simulink subsystem "motores"  (R2023b)
settings: Solver=VariableStepAuto  StartTime=0.0  StopTime=10.0  RelTol=1e-3
libraries: arduinolib x6, simulink x2
settings Model: Creator=Usuario_UMA  LastModifiedBy=Manuel

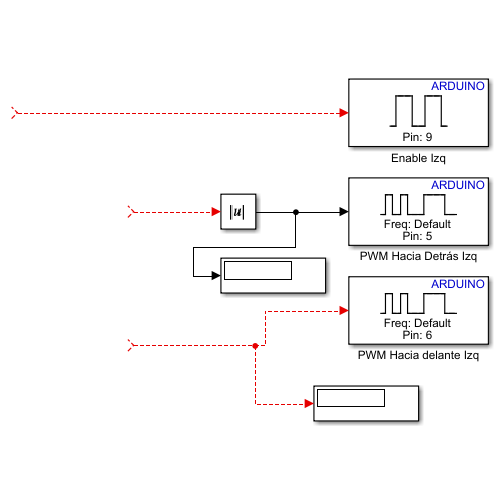
[thumbnail: Simulink's stored preview of the top-level diagram]
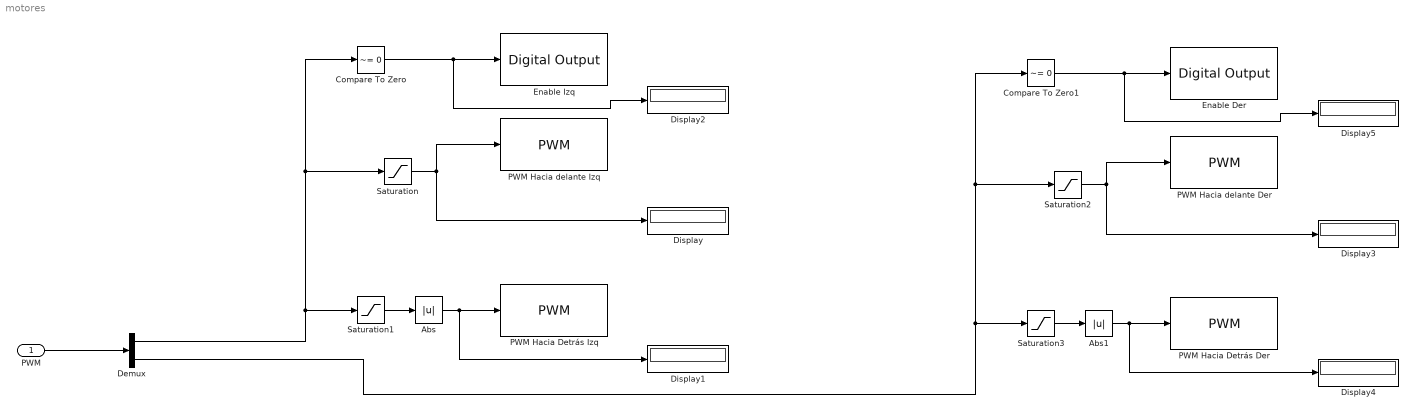
== system motores ==
  PWM : Inport
  Abs : Abs  SaturateOnIntegerOverflow=off
  Abs1 : Abs  SaturateOnIntegerOverflow=off
  Compare To Zero : simulink/Logic and Bit Operations/Compare To Zero  relop=~=  OutDataTypeStr=boolean
  Compare To Zero1 : simulink/Logic and Bit Operations/Compare To Zero  relop=~=  OutDataTypeStr=boolean
  Demux : Demux  Outputs=2
  Display{,1..5} (6 alike) : Display
  Enable Der : arduinolib/Digital Output  pinNumber=12  Direction=output  blockPlatform=arduino
  Enable Izq : arduinolib/Digital Output  pinNumber=13  Direction=output  blockPlatform=arduino
  PWM Hacia Detrás Der : arduinolib/PWM  pinNumber=4  frequencyType=Default  desiredFrequency=490.2  achievableFrequency=490.2
  PWM Hacia Detrás Izq : arduinolib/PWM  pinNumber=7  frequencyType=Default  desiredFrequency=490.2  achievableFrequency=490.2
  PWM Hacia delante Der : arduinolib/PWM  pinNumber=5  frequencyType=Default  desiredFrequency=490.2  achievableFrequency=490.2
  PWM Hacia delante Izq : arduinolib/PWM  pinNumber=6  frequencyType=Default  desiredFrequency=490.2  achievableFrequency=490.2
  Saturation : Saturate  UpperLimit=255  LowerLimit=1
  Saturation1 : Saturate  UpperLimit=0  LowerLimit=-255
  Saturation2 : Saturate  UpperLimit=255  LowerLimit=1
  Saturation3 : Saturate  UpperLimit=1  LowerLimit=-255
  wires:
  Abs/1 -> Display1/1, PWM Hacia Detrás Izq/1
  PWM/1 -> Demux/1
  Compare To Zero/1 -> Enable Izq/1, Display2/1
  Saturation/1 -> Display/1, PWM Hacia delante Izq/1
  Saturation1/1 -> Abs/1
  Abs1/1 -> Display4/1, PWM Hacia Detrás Der/1
  Compare To Zero1/1 -> Enable Der/1, Display5/1
  Saturation2/1 -> Display3/1, PWM Hacia delante Der/1
  Saturation3/1 -> Abs1/1
  Demux/2 -> Compare To Zero1/1, Saturation2/1, Saturation3/1
  Demux/1 -> Compare To Zero/1, Saturation/1, Saturation1/1
